simulink model "Problem8"  (R2020a)
settings: Solver=VariableStepAuto  StartTime=0.0  StopTime=inf  RelTol=1e-3
settings Model: Creator=shweta  LastModifiedBy=shweta

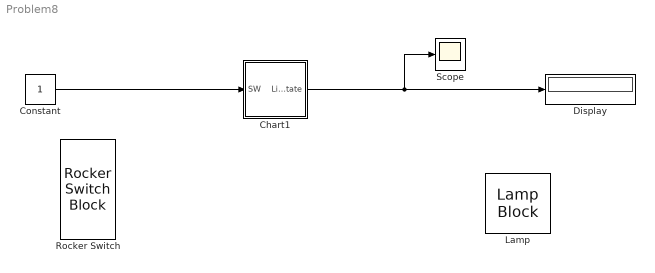
== system Problem8 ==
  Chart1 : Stateflow chart  TreatAsAtomicUnit=on
  Constant : Constant
  Display : Display
  Lamp : LampBlock
  Rocker Switch : RockerSwitchBlock
      settings: Values={{'Off', 'On'}, [0 1]}
  Scope : Scope
  wires:
  Constant/1 -> Chart1/1(SW)
  Chart1/1(LightState) -> Scope/1, Display/1

== stateflow chart Problem8/Chart1 ==
  state off
    entry:
    LightState=0;
  state on
    entry:
    LightState=1;
  (default) -> off
  off -> on : [SW==1]
  on -> off : [SW==0]
  data: SW input; LightState output
